simulink model "Control_test"  (R2014b)
settings: Solver=FixedStepDiscrete  StartTime=0.0  StopTime=Inf  FixedStep=0.001  RelTol=1e-3
PostLoadFcn:
  | , if any(exist('dsrtsu_mdlpostloadfcn', 'file') == [2, 3, 6]), try dsrtsu_mdlpostloadfcn('Execute', bdroot); catch fprintf('Error in PostLoadFcn (dsrtsu_mdlpostloadfcn) for model "%s":\n %s\n', bdroot, lasterr); end, end,
undefined symbols (not defined in the file or in its folder): dtLocal, slcm
libraries: rtican x163, simulink x14
(part 33 of 34)

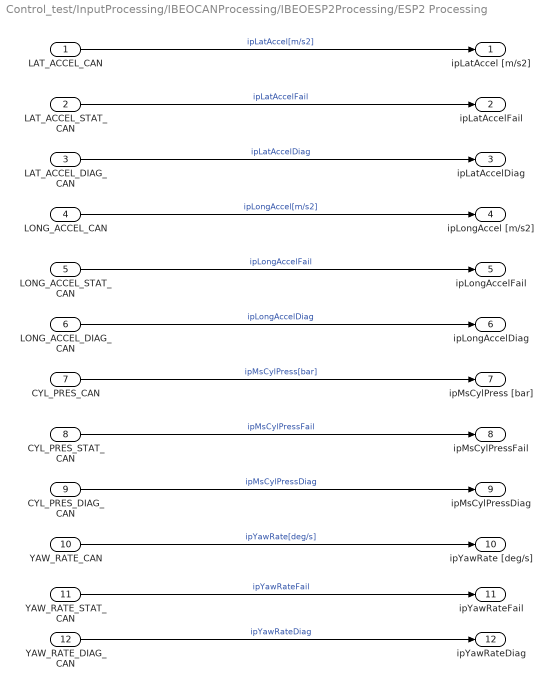
== system Control_test/InputProcessing/IBEOCANProcessing/IBEOESP2Processing/ESP2 Processing ==
  LAT_ACCEL_CAN : Inport
  LAT_ACCEL_STAT_CAN : Inport  Port=2
  LAT_ACCEL_DIAG_CAN : Inport  Port=3
  LONG_ACCEL_CAN : Inport  Port=4
  LONG_ACCEL_STAT_CAN : Inport  Port=5
  LONG_ACCEL_DIAG_CAN : Inport  Port=6
  CYL_PRES_CAN : Inport  Port=7
  CYL_PRES_STAT_CAN : Inport  Port=8
  CYL_PRES_DIAG_CAN : Inport  Port=9
  YAW_RATE_CAN : Inport  Port=10
  YAW_RATE_STAT_CAN : Inport  Port=11
  YAW_RATE_DIAG_CAN : Inport  Port=12
  ipLatAccel [m/s2] : Outport
  ipLatAccelFail : Outport  Port=2
  ipLatAccelDiag : Outport  Port=3
  ipLongAccel [m/s2] : Outport  Port=4
  ipLongAccelFail : Outport  Port=5
  ipLongAccelDiag : Outport  Port=6
  ipMsCylPress [bar] : Outport  Port=7
  ipMsCylPressFail : Outport  Port=8
  ipMsCylPressDiag : Outport  Port=9
  ipYawRate [deg/s] : Outport  Port=10
  ipYawRateFail : Outport  Port=11
  ipYawRateDiag : Outport  Port=12
  wires:
  YAW_RATE_CAN/1 -> ipYawRate [deg/s]/1  "ipYawRate[deg/s]"
  LONG_ACCEL_CAN/1 -> ipLongAccel [m/s2]/1  "ipLongAccel[m/s2]"
  LAT_ACCEL_STAT_CAN/1 -> ipLatAccelFail/1  "ipLatAccelFail"
  LAT_ACCEL_DIAG_CAN/1 -> ipLatAccelDiag/1  "ipLatAccelDiag"
  LONG_ACCEL_STAT_CAN/1 -> ipLongAccelFail/1  "ipLongAccelFail"
  LONG_ACCEL_DIAG_CAN/1 -> ipLongAccelDiag/1  "ipLongAccelDiag"
  CYL_PRES_CAN/1 -> ipMsCylPress [bar]/1  "ipMsCylPress[bar]"
  CYL_PRES_STAT_CAN/1 -> ipMsCylPressFail/1  "ipMsCylPressFail"
  CYL_PRES_DIAG_CAN/1 -> ipMsCylPressDiag/1  "ipMsCylPressDiag"
  YAW_RATE_STAT_CAN/1 -> ipYawRateFail/1  "ipYawRateFail"
  YAW_RATE_DIAG_CAN/1 -> ipYawRateDiag/1  "ipYawRateDiag"
  LAT_ACCEL_CAN/1 -> ipLatAccel [m/s2]/1  "ipLatAccel[m/s2]"

== system Control_test/InputProcessing/IBEOCANProcessing/IBEOSASProcessing/SAS1 Processing ==
  SAS_Angle_CAN : Inport
  SAS_Speed_CAN : Inport  Port=2
  MsgCount_CAN : Inport  Port=3
  CheckSum_CAN : Inport  Port=4
  Add2 : Sum  Inputs=+-
  Compare To Constant1 : simulink/Logic and Bit Operations/Compare To Constant  relop=<=  const=3276.7  OutDataTypeStr=boolean  ZeroCross=off
  Constant6 : Constant  Value=6553.6  SampleTime=Inf
  ErrProcessing1 : Subsystem
  ErrProcessing2 : Subsystem
  Switch1 : Switch  Criteria=u2 > Threshold
  ipStrAng [deg] : Outport
  ipStrAngEr : Outport  Port=2
  ipStrSpd [deg/s] : Outport  Port=3
  ipStrSpdEr : Outport  Port=4
  ipSasCnt : Outport  Port=5
  ipSasCksum : Outport  Port=6
  wires:
  SAS_Speed_CAN/1 -> ErrProcessing1/1(In1)
  Add2/1 -> Switch1/3
  Constant6/1 -> Add2/2
  Compare To Constant1/1 -> Switch1/2
  Switch1/1 -> ipStrAng [deg]/1  "ipStrAng[deg]"
  ErrProcessing2/2(ErrFlag) -> ipStrAngEr/1  "ipStrAngEr"
  ErrProcessing1/2(ErrFlag) -> ipStrSpdEr/1  "ipStrSpdEr"
  ErrProcessing1/1(Data) -> ipStrSpd [deg/s]/1  "ipStrSpd[deg/s]"
  MsgCount_CAN/1 -> ipSasCnt/1  "ipSasCnt"
  CheckSum_CAN/1 -> ipSasCksum/1  "ipSasCksum"
  SAS_Angle_CAN/1 -> ErrProcessing2/1(In1)
  ErrProcessing2/1(Data) -> Compare To Constant1/1, Switch1/1, Add2/1

== system Control_test/InputProcessing/RadarCanProcessing/Primary Target Selection/Default ==
  Bus Creator : BusCreator  Inputs=12
  Constant : Constant  Value=255  SampleTime=0.01
  Out1 : Outport
  wires:
  Bus Creator/1 -> Out1/1  "NoTrack"
  Constant/1 -> Bus Creator/1, Bus Creator/2, Bus Creator/3, Bus Creator/4, Bus Creator/5, Bus Creator/6, Bus Creator/7, Bus Creator/8, Bus Creator/9, Bus Creator/10, Bus Creator/11, Bus Creator/12

== system Control_test/InputProcessing/VehicleCanProcessing/CLU2Processing/CLU2Processing ==
  CF_Clu_TrunSigLh_CAN : Inport
  CF_Clu_TurnSigRh_CAN : Inport  Port=2
  ipCluTurnSigLh : Outport
  ipCluTurnSigRh : Outport  Port=2
  wires:
  CF_Clu_TrunSigLh_CAN/1 -> ipCluTurnSigLh/1  "ipCluTurnSigLh"
  CF_Clu_TurnSigRh_CAN/1 -> ipCluTurnSigRh/1  "ipCluTurnSigRh"

== system Control_test/InputProcessing/VehicleCanProcessing/EMS1Processing/EMS1 Processing ==
  VS_CAN : Inport
  ErrProcessing : Subsystem
  ipEmsVehSpd [kph] : Outport
  ipEmsVehSpdFail : Outport  Port=2
  wires:
  VS_CAN/1 -> ErrProcessing/1(In1)
  ErrProcessing/1(Data) -> ipEmsVehSpd [kph]/1  "ipEmsVehSpd[kph]"
  ErrProcessing/2(ErrFlag) -> ipEmsVehSpdFail/1  "ipEmsVehSpdFail"

== system Control_test/InputProcessing/VehicleCanProcessing/ESP2Processing/ESP2 Processing ==
  LAT_ACCEL_CAN : Inport
  LAT_ACCEL_STAT_CAN : Inport  Port=2
  LAT_ACCEL_DIAG_CAN : Inport  Port=3
  LONG_ACCEL_CAN : Inport  Port=4
  LONG_ACCEL_STAT_CAN : Inport  Port=5
  LONG_ACCEL_DIAG_CAN : Inport  Port=6
  CYL_PRES_CAN : Inport  Port=7
  CYL_PRES_STAT_CAN : Inport  Port=8
  CYL_PRES_DIAG_CAN : Inport  Port=9
  YAW_RATE_CAN : Inport  Port=10
  YAW_RATE_STAT_CAN : Inport  Port=11
  YAW_RATE_DIAG_CAN : Inport  Port=12
  ipLatAccel [m/s2] : Outport
  ipLatAccelFail : Outport  Port=2
  ipLatAccelDiag : Outport  Port=3
  ipLongAccel [m/s2] : Outport  Port=4
  ipLongAccelFail : Outport  Port=5
  ipLongAccelDiag : Outport  Port=6
  ipMsCylPress [bar] : Outport  Port=7
  ipMsCylPressFail : Outport  Port=8
  ipMsCylPressDiag : Outport  Port=9
  ipYawRate [deg/s] : Outport  Port=10
  ipYawRateFail : Outport  Port=11
  ipYawRateDiag : Outport  Port=12
  wires:
  YAW_RATE_CAN/1 -> ipYawRate [deg/s]/1  "ipYawRate[deg/s]"
  LONG_ACCEL_CAN/1 -> ipLongAccel [m/s2]/1  "ipLongAccel[m/s2]"
  LAT_ACCEL_STAT_CAN/1 -> ipLatAccelFail/1  "ipLatAccelFail"
  LAT_ACCEL_DIAG_CAN/1 -> ipLatAccelDiag/1  "ipLatAccelDiag"
  LONG_ACCEL_STAT_CAN/1 -> ipLongAccelFail/1  "ipLongAccelFail"
  LONG_ACCEL_DIAG_CAN/1 -> ipLongAccelDiag/1  "ipLongAccelDiag"
  CYL_PRES_CAN/1 -> ipMsCylPress [bar]/1  "ipMsCylPress[bar]"
  CYL_PRES_STAT_CAN/1 -> ipMsCylPressFail/1  "ipMsCylPressFail"
  CYL_PRES_DIAG_CAN/1 -> ipMsCylPressDiag/1  "ipMsCylPressDiag"
  YAW_RATE_STAT_CAN/1 -> ipYawRateFail/1  "ipYawRateFail"
  YAW_RATE_DIAG_CAN/1 -> ipYawRateDiag/1  "ipYawRateDiag"
  LAT_ACCEL_CAN/1 -> ipLatAccel [m/s2]/1  "ipLatAccel[m/s2]"

== system Control_test/InputProcessing/VehicleCanProcessing/MDPS3Processing/MDPS3 Processing ==
  CR_Mdps_StrColTq_CAN : Inport
  CR_Mdps_ToiUnavail_CAN : Inport  Port=2
  CR_Mdps_ToiActive_CAN : Inport  Port=3
  CR_Mdps_ToiFit_CAN : Inport  Port=4
  CR_Mdps_FailStat_CAN : Inport  Port=5
  ipMdpsStrColTq : Outport
  ipMdpsToiUnavail : Outport  Port=2
  ipMdpsToiActive : Outport  Port=3
  ipMdpsToiFit : Outport  Port=4
  ipMdpsFailStat : Outport  Port=5
  wires:
  CR_Mdps_FailStat_CAN/1 -> ipMdpsFailStat/1  "ipMdpsFailStat"
  CR_Mdps_ToiActive_CAN/1 -> ipMdpsToiActive/1  "ipMdpsToiActive"
  CR_Mdps_ToiUnavail_CAN/1 -> ipMdpsToiUnavail/1  "ipMdpsToiUnavail"
  CR_Mdps_StrColTq_CAN/1 -> ipMdpsStrColTq/1  "ipMdpsStrColTq"
  CR_Mdps_ToiFit_CAN/1 -> ipMdpsToiFit/1  "ipMdpsToiFit"

== system Control_test/InputProcessing/VehicleCanProcessing/SAS1Processing/SAS1 Processing ==
  SAS_Angle_CAN : Inport
  SAS_Speed_CAN : Inport  Port=2
  MsgCount_CAN : Inport  Port=3
  CheckSum_CAN : Inport  Port=4
  Add2 : Sum  Inputs=+-
  Compare To Constant1 : simulink/Logic and Bit Operations/Compare To Constant  relop=<=  const=3276.7  OutDataTypeStr=uint8  ZeroCross=off
  Constant6 : Constant  Value=6553.6  SampleTime=Inf
  ErrProcessing1 : Subsystem
  ErrProcessing2 : Subsystem
  Switch1 : Switch  Criteria=u2 > Threshold
  ipStrAng [deg] : Outport
  ipStrAngEr : Outport  Port=2
  ipStrSpd [deg/s] : Outport  Port=3
  ipStrSpdEr : Outport  Port=4
  ipSasCnt : Outport  Port=5
  ipSasCksum : Outport  Port=6
  wires:
  SAS_Speed_CAN/1 -> ErrProcessing1/1(In1)
  Add2/1 -> Switch1/3
  Constant6/1 -> Add2/2
  Compare To Constant1/1 -> Switch1/2
  Switch1/1 -> ipStrAng [deg]/1  "ipStrAng[deg]"
  ErrProcessing2/2(ErrFlag) -> ipStrAngEr/1  "ipStrAngEr"
  ErrProcessing1/2(ErrFlag) -> ipStrSpdEr/1  "ipStrSpdEr"
  ErrProcessing1/1(Data) -> ipStrSpd [deg/s]/1  "ipStrSpd[deg/s]"
  MsgCount_CAN/1 -> ipSasCnt/1  "ipSasCnt"
  CheckSum_CAN/1 -> ipSasCksum/1  "ipSasCksum"
  SAS_Angle_CAN/1 -> ErrProcessing2/1(In1)
  ErrProcessing2/1(Data) -> Compare To Constant1/1, Switch1/1, Add2/1

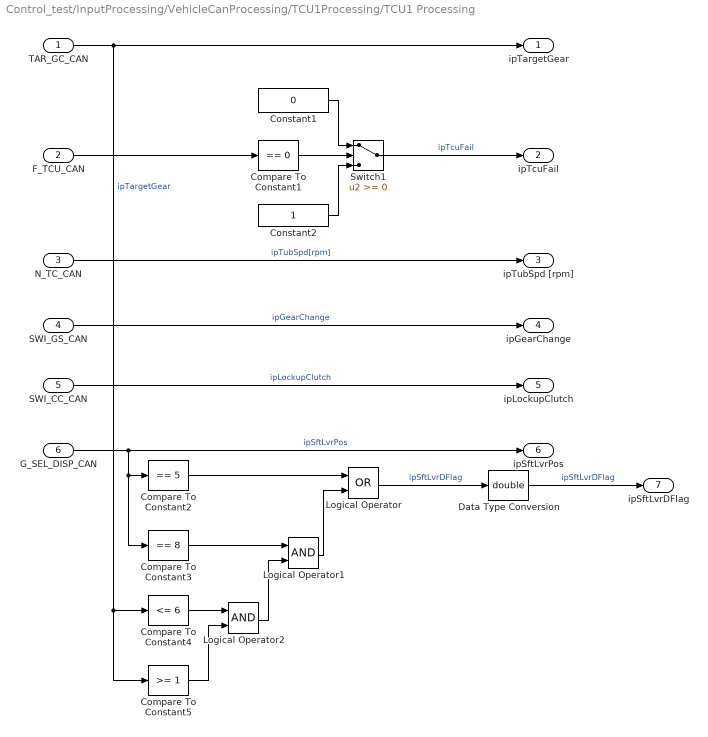
== system Control_test/InputProcessing/VehicleCanProcessing/TCU1Processing/TCU1 Processing ==
  TAR_GC_CAN : Inport
  F_TCU_CAN : Inport  Port=2
  N_TC_CAN : Inport  Port=3
  SWI_GS_CAN : Inport  Port=4
  SWI_CC_CAN : Inport  Port=5
  G_SEL_DISP_CAN : Inport  Port=6
  Compare To Constant1 : simulink/Logic and Bit Operations/Compare To Constant  relop===  const=0  OutDataTypeStr=uint8  ZeroCross=off
  Compare To Constant2 : simulink/Logic and Bit Operations/Compare To Constant  relop===  const=5  OutDataTypeStr=uint8  ZeroCross=off
  Compare To Constant3 : simulink/Logic and Bit Operations/Compare To Constant  relop===  const=8  OutDataTypeStr=uint8  ZeroCross=off
  Compare To Constant4 : simulink/Logic and Bit Operations/Compare To Constant  relop=<=  const=6  OutDataTypeStr=uint8  ZeroCross=off
  Compare To Constant5 : simulink/Logic and Bit Operations/Compare To Constant  relop=>=  const=1  OutDataTypeStr=uint8  ZeroCross=off
  Constant1 : Constant  Value=0  SampleTime=Inf
  Constant2 : Constant  SampleTime=Inf
  Data Type Conversion : DataTypeConversion  OutDataTypeStr=double
  Logical Operator : Logic  Operator=OR  AllPortsSameDT=off  OutDataTypeStr=boolean
  Logical Operator1 : Logic  AllPortsSameDT=off  OutDataTypeStr=boolean
  Logical Operator2 : Logic  AllPortsSameDT=off  OutDataTypeStr=boolean
  Switch1 : Switch
  ipTargetGear : Outport
  ipTcuFail : Outport  Port=2
  ipTubSpd [rpm] : Outport  Port=3
  ipGearChange : Outport  Port=4
  ipLockupClutch : Outport  Port=5
  ipSftLvrPos : Outport  Port=6
  ipSftLvrDFlag : Outport  Port=7
  wires:
  Compare To Constant5/1 -> Logical Operator2/2
  Logical Operator2/1 -> Logical Operator1/2
  Compare To Constant4/1 -> Logical Operator2/1
  Logical Operator1/1 -> Logical Operator/2
  Compare To Constant3/1 -> Logical Operator1/1
  Logical Operator/1 -> Data Type Conversion/1  "ipSftLvrDFlag"
  Compare To Constant2/1 -> Logical Operator/1
  G_SEL_DISP_CAN/1 -> Compare To Constant3/1, Compare To Constant2/1, ipSftLvrPos/1  "ipSftLvrPos"
  SWI_CC_CAN/1 -> ipLockupClutch/1  "ipLockupClutch"
  SWI_GS_CAN/1 -> ipGearChange/1  "ipGearChange"
  N_TC_CAN/1 -> ipTubSpd [rpm]/1  "ipTubSpd[rpm]"
  Switch1/1 -> ipTcuFail/1  "ipTcuFail"
  Constant2/1 -> Switch1/3
  Constant1/1 -> Switch1/1
  Compare To Constant1/1 -> Switch1/2
  F_TCU_CAN/1 -> Compare To Constant1/1
  TAR_GC_CAN/1 -> Compare To Constant5/1, Compare To Constant4/1, ipTargetGear/1  "ipTargetGear"
  Data Type Conversion/1 -> ipSftLvrDFlag/1  "ipSftLvrDFlag"

== system Control_test/InputProcessing/VehicleCanProcessing/WhlSpdProcessing/WhlSpd Processing ==
  WHL_SPD_FL_CAN : Inport
  WHL_SPD_FR_CAN : Inport  Port=2
  WHL_SPD_RL_CAN : Inport  Port=3
  WHL_SPD_RR_CAN : Inport  Port=4
  Add2 : Sum
  Constant3 : Constant  Value=2  SampleTime=Inf
  ErrProcessing : Subsystem
  ErrProcessing1 : Subsystem
  ErrProcessing2 : Subsystem
  ErrProcessing3 : Subsystem
  Gain : Gain  Gain=1/3.6
  Product5 : Product  Inputs=*/
  ipWhlSpdFl [kph] : Outport
  ipWhlSpdFlEr : Outport  Port=2
  ipWhlSpdFr [kph] : Outport  Port=3
  ipWhlSpdFrEr : Outport  Port=4
  ipWhlSpdRl [kph] : Outport  Port=5
  ipWhlSpdRlEr : Outport  Port=6
  ipWhlSpdRr [kph] : Outport  Port=7
  ipWhlSpdRrEr : Outport  Port=8
  ipVehSpdWhl [kph] : Outport  Port=9
  ipVehSpdWhl [m/s] : Outport  Port=10
  wires:
  Gain/1 -> ipVehSpdWhl [m/s]/1  "ipVehSpdWhl[m/s]"
  Constant3/1 -> Product5/2
  Add2/1 -> Product5/1
  WHL_SPD_FR_CAN/1 -> ErrProcessing1/1(In1)
  WHL_SPD_FL_CAN/1 -> ErrProcessing/1(In1)
  ErrProcessing/1(Data) -> Add2/1, ipWhlSpdFl [kph]/1  "ipWhlSpdFl[kph]"
  ErrProcessing/2(ErrFlag) -> ipWhlSpdFlEr/1  "ipWhlSpdFlEr"
  ErrProcessing1/1(Data) -> Add2/2, ipWhlSpdFr [kph]/1  "ipWhlSpdFr[kph]"
  ErrProcessing1/2(ErrFlag) -> ipWhlSpdFrEr/1  "ipWhlSpdFrEr"
  WHL_SPD_RL_CAN/1 -> ErrProcessing2/1(In1)
  ErrProcessing2/1(Data) -> ipWhlSpdRl [kph]/1  "ipWhlSpdRl[kph]"
  ErrProcessing2/2(ErrFlag) -> ipWhlSpdRlEr/1  "ipWhlSpdRlEr"
  WHL_SPD_RR_CAN/1 -> ErrProcessing3/1(In1)
  ErrProcessing3/1(Data) -> ipWhlSpdRr [kph]/1  "ipWhlSpdRr[kph]"
  ErrProcessing3/2(ErrFlag) -> ipWhlSpdRrEr/1  "ipWhlSpdRrEr"
  Product5/1 -> ipVehSpdWhl [kph]/1, Gain/1  "ipVehSpdWhl[kph]"

== system Control_test/OutputProcessing/RadarCanProcessing/Transmit Radar Msg 0x4F0/If Action Subsystem ==
  In1 : Inport
  Action Port : ActionPort  ActionType=then
  Out1 : Outport
  wires:
  In1/1 -> Out1/1

== system Control_test/OutputProcessing/RadarCanProcessing/Transmit Radar Msg 0x4F0/If Action Subsystem1 ==
  In1 : Inport
  Action Port : ActionPort  ActionType=else
  Out1 : Outport
  wires:
  In1/1 -> Out1/1

== system Control_test/OutputProcessing/VehicleCanProcessing/LKAS2/Angle 2 Torque ==
  ISAS_Cmd(deg) : Inport
  ControlOn : Inport  Port=2
  Vs : Inport  Port=3
  SteeringAngle : Inport  Port=4
  IGainSpeed : Gain
  I_gain_spd : Constant  Value=500
  PGainSAS : Gain
  PGainSpeed : Gain
  PI controller : Subsystem
  P_gain_sas_map : Lookup  InputValues=[0,30,60,80,100]  Table=[170,170,300,300,330]  LookUpMeth=Interpolation-Use End Values
  P_gain_spd_map : Lookup  InputValues=[0,30,60,80,100]  Table=[300,300,400,400,450]  LookUpMeth=Interpolation-Use End Values
  Rate Limiter steering : RateLimiter  RisingSlewLimit=50  FallingSlewLimit=-50  SampleTimeMode=inherited
  Saturation steering torque : Saturate  UpperLimit=7.5  LowerLimit=-7.5
  Steering TQ : Outport
  wires:
  I_gain_spd/1 -> IGainSpeed/1
  ControlOn/1 -> PI controller/1(Active_flag)  "ActiveFlag"
  ISAS_Cmd(deg)/1 -> PI controller/2(SAS_Cmd(deg))  "SAS_Cmd"
  SteeringAngle/1 -> PI controller/3(SAS_Angle(deg))
  Saturation steering torque/1 -> Rate Limiter steering/1  "Tq_after_sat"
  Rate Limiter steering/1 -> Steering TQ/1  "Control Tq"
  Vs/1 -> P_gain_spd_map/1, P_gain_sas_map/1
  PI controller/1(Tq) -> Saturation steering torque/1  "Tq_before_sat"
  P_gain_sas_map/1 -> PGainSAS/1
  P_gain_spd_map/1 -> PGainSpeed/1
  PGainSpeed/1 -> PI controller/5(P_gain_spd)  "PGainSpeed"
  PGainSAS/1 -> PI controller/4(P_gain_sas)  "PGainSAS"
  IGainSpeed/1 -> PI controller/6(I_gain_spd)

== system Control_test/OutputProcessing/VehicleCanProcessing/LKAS2/TxLKAS2CAN ==
  Tq : Inport
  ActiveFlag_Out : Inport  Port=2
  TOI_Fault : Inport  Port=3
  MessageCounter : Subsystem  mask(Rolling Counter){cyc_time=20, calc_time=2, n_bit=4}
      mask prompts: cyc_time "Cyclic Time (ms)"; calc_time "Model loop time [ms]"; n_bit "Number of bits"
      mask help: This block is a rolling counter that overflows back to zero after it has been the maximum value for the specified number of bits.
  Tx_ADAS_data : Subsystem
  Checksum_Out : Outport
  LKAS_Tq_Out : Outport  Port=2
  MessageCounter_Out : Outport  Port=3
  TOI_Fault_Out : Outport  Port=4
  ActiveTOI_Out : Outport  Port=5
  wires:
  MessageCounter/1(Counter) -> Tx_ADAS_data/1(MessageCounter)
  Tx_ADAS_data/1(LKAS_Toq_Out) -> LKAS_Tq_Out/1
  Tq/1 -> Tx_ADAS_data/2(SteeringTorqueRuest)
  ActiveFlag_Out/1 -> Tx_ADAS_data/3(ActiveTOI)
  Tx_ADAS_data/4(MessageCounter_Out) -> MessageCounter_Out/1
  Tx_ADAS_data/2(ActiveTOI_Out) -> ActiveTOI_Out/1
  TOI_Fault/1 -> Tx_ADAS_data/4(TOI_Fault)
  Tx_ADAS_data/3(TOI_Fault_Out) -> TOI_Fault_Out/1
  Tx_ADAS_data/5(Checksum_Out) -> Checksum_Out/1

== system Control_test/RTI Data/RTI Data Store/RTI Data Store/RTI Data Store ==
  RTI Data Store : Subsystem  mask(RTI_DATA_STORE){}
      mask help:
      | RTI Data Store Block. This block is used by RTI to store internal model dependent data. Deleting this block will result in data loss.
      |
      | NEVER DELETE, COPY, OR MODIFY THIS BLOCK!
      mask Help:
      | RTI Data Store Block. This block is used by RTI to store internal model dependent data. Deleting this block will result in data loss.
      | 
      | NEVER DELETE, COPY, OR MODIFY THIS BLOCK!
      mask Display: text(0.5, 0.5, ' ', 'HorizontalAlignment', 'center');

== system Control_test/InputProcessing/IBEOCANProcessing/IBEOSASProcessing/SAS1 Processing/ErrProcessing1 ==
  In1 : Inport
  If : If  NumInputs=2  IfExpression=u1 == 1020 & u2>1  ElseIfExpressions=u1 == 1020 & u2<=1
  If Action Subsystem : Subsystem  TreatAsAtomicUnit=on
  If Action Subsystem1 : Subsystem  TreatAsAtomicUnit=on
  If Action Subsystem2 : Subsystem  TreatAsAtomicUnit=on
  Memory : Memory
  Memory1 : Memory
  Merge : Merge  Inputs=3
  Merge1 : Merge  Inputs=3
  Merge2 : Merge  Inputs=3
  Data : Outport
  ErrFlag : Outport  Port=2
  wires:
  In1/1 -> If/1, If Action Subsystem1/1(In1)
  If/1 -> If Action Subsystem/Action
  If/3 -> If Action Subsystem1/Action
  If/2 -> If Action Subsystem2/Action
  If Action Subsystem/1(Data) -> Merge/1
  If Action Subsystem2/1(Data) -> Merge/2
  If Action Subsystem1/1(Data) -> Merge/3
  Merge/1 -> Data/1, Memory1/1
  Memory1/1 -> If Action Subsystem2/1(In1)
  If Action Subsystem/2(Count) -> Merge1/1
  If Action Subsystem2/2(Count) -> Merge1/2
  If Action Subsystem1/2(Count) -> Merge1/3
  Merge1/1 -> Memory/1
  Memory/1 -> If Action Subsystem/1(In1), If/2, If Action Subsystem2/2(In2)
  If Action Subsystem/3(Flag) -> Merge2/1
  If Action Subsystem2/3(Flag) -> Merge2/2
  If Action Subsystem1/3(Flag) -> Merge2/3
  Merge2/1 -> ErrFlag/1

== system Control_test/InputProcessing/IBEOCANProcessing/IBEOSASProcessing/SAS1 Processing/ErrProcessing2 ==
  In1 : Inport
  If : If  NumInputs=2  IfExpression=u1 == 3276.7 & u2>1  ElseIfExpressions=u1 == 3276.7 & u2<=1
  If Action Subsystem : Subsystem  TreatAsAtomicUnit=on
  If Action Subsystem1 : Subsystem  TreatAsAtomicUnit=on
  If Action Subsystem2 : Subsystem  TreatAsAtomicUnit=on
  Memory : Memory
  Memory1 : Memory
  Merge : Merge  Inputs=3
  Merge1 : Merge  Inputs=3
  Merge2 : Merge  Inputs=3
  Data : Outport
  ErrFlag : Outport  Port=2
  wires:
  Merge2/1 -> ErrFlag/1
  If Action Subsystem1/3(Flag) -> Merge2/3
  If Action Subsystem2/3(Flag) -> Merge2/2
  If Action Subsystem/3(Flag) -> Merge2/1
  Memory/1 -> If Action Subsystem2/2(In2), If/2, If Action Subsystem/1(In1)
  Merge1/1 -> Memory/1
  If Action Subsystem1/2(Count) -> Merge1/3
  If Action Subsystem2/2(Count) -> Merge1/2
  If Action Subsystem/2(Count) -> Merge1/1
  Memory1/1 -> If Action Subsystem2/1(In1)
  Merge/1 -> Memory1/1, Data/1
  If Action Subsystem1/1(Data) -> Merge/3
  If Action Subsystem2/1(Data) -> Merge/2
  If Action Subsystem/1(Data) -> Merge/1
  If/2 -> If Action Subsystem2/Action
  If/3 -> If Action Subsystem1/Action
  If/1 -> If Action Subsystem/Action
  In1/1 -> If Action Subsystem1/1(In1), If/1

== system Control_test/InputProcessing/VehicleCanProcessing/EMS1Processing/EMS1 Processing/ErrProcessing ==
  In1 : Inport
  If : If  NumInputs=2  IfExpression=u1 == 255 & u2>1  ElseIfExpressions=u1 == 255 & u2<=1
  If Action Subsystem : Subsystem  TreatAsAtomicUnit=on
  If Action Subsystem1 : Subsystem  TreatAsAtomicUnit=on
  If Action Subsystem2 : Subsystem  TreatAsAtomicUnit=on
  Memory : Memory
  Memory1 : Memory
  Merge : Merge  Inputs=3
  Merge1 : Merge  Inputs=3
  Merge2 : Merge  Inputs=3
  Data : Outport
  ErrFlag : Outport  Port=2
  wires:
  In1/1 -> If/1, If Action Subsystem1/1(In1)
  If/1 -> If Action Subsystem/Action
  If/3 -> If Action Subsystem1/Action
  If/2 -> If Action Subsystem2/Action
  If Action Subsystem/1(Data) -> Merge/1
  If Action Subsystem2/1(Data) -> Merge/2
  If Action Subsystem1/1(Data) -> Merge/3
  Merge/1 -> Data/1, Memory1/1
  Memory1/1 -> If Action Subsystem2/1(In1)
  If Action Subsystem/2(Count) -> Merge1/1
  If Action Subsystem2/2(Count) -> Merge1/2
  If Action Subsystem1/2(Count) -> Merge1/3
  Merge1/1 -> Memory/1
  Memory/1 -> If Action Subsystem/1(In1), If/2, If Action Subsystem2/2(In2)
  If Action Subsystem/3(Flag) -> Merge2/1
  If Action Subsystem2/3(Flag) -> Merge2/2
  If Action Subsystem1/3(Flag) -> Merge2/3
  Merge2/1 -> ErrFlag/1

== system Control_test/InputProcessing/VehicleCanProcessing/SAS1Processing/SAS1 Processing/ErrProcessing1 ==
  In1 : Inport
  If : If  NumInputs=2  IfExpression=u1 == 1020 & u2>1  ElseIfExpressions=u1 == 1020 & u2<=1
  If Action Subsystem : Subsystem  TreatAsAtomicUnit=on
  If Action Subsystem1 : Subsystem  TreatAsAtomicUnit=on
  If Action Subsystem2 : Subsystem  TreatAsAtomicUnit=on
  Memory : Memory
  Memory1 : Memory
  Merge : Merge  Inputs=3
  Merge1 : Merge  Inputs=3
  Merge2 : Merge  Inputs=3
  Data : Outport
  ErrFlag : Outport  Port=2
  wires:
  In1/1 -> If/1, If Action Subsystem1/1(In1)
  If/1 -> If Action Subsystem/Action
  If/3 -> If Action Subsystem1/Action
  If/2 -> If Action Subsystem2/Action
  If Action Subsystem/1(Data) -> Merge/1
  If Action Subsystem2/1(Data) -> Merge/2
  If Action Subsystem1/1(Data) -> Merge/3
  Merge/1 -> Data/1, Memory1/1
  Memory1/1 -> If Action Subsystem2/1(In1)
  If Action Subsystem/2(Count) -> Merge1/1
  If Action Subsystem2/2(Count) -> Merge1/2
  If Action Subsystem1/2(Count) -> Merge1/3
  Merge1/1 -> Memory/1
  Memory/1 -> If Action Subsystem/1(In1), If/2, If Action Subsystem2/2(In2)
  If Action Subsystem/3(Flag) -> Merge2/1
  If Action Subsystem2/3(Flag) -> Merge2/2
  If Action Subsystem1/3(Flag) -> Merge2/3
  Merge2/1 -> ErrFlag/1

== system Control_test/InputProcessing/VehicleCanProcessing/SAS1Processing/SAS1 Processing/ErrProcessing2 ==
  In1 : Inport
  If : If  NumInputs=2  IfExpression=u1 == 3276.7 & u2>1  ElseIfExpressions=u1 == 3276.7 & u2<=1
  If Action Subsystem : Subsystem  TreatAsAtomicUnit=on
  If Action Subsystem1 : Subsystem  TreatAsAtomicUnit=on
  If Action Subsystem2 : Subsystem  TreatAsAtomicUnit=on
  Memory : Memory
  Memory1 : Memory
  Merge : Merge  Inputs=3
  Merge1 : Merge  Inputs=3
  Merge2 : Merge  Inputs=3
  Data : Outport
  ErrFlag : Outport  Port=2
  wires:
  Merge2/1 -> ErrFlag/1
  If Action Subsystem1/3(Flag) -> Merge2/3
  If Action Subsystem2/3(Flag) -> Merge2/2
  If Action Subsystem/3(Flag) -> Merge2/1
  Memory/1 -> If Action Subsystem2/2(In2), If/2, If Action Subsystem/1(In1)
  Merge1/1 -> Memory/1
  If Action Subsystem1/2(Count) -> Merge1/3
  If Action Subsystem2/2(Count) -> Merge1/2
  If Action Subsystem/2(Count) -> Merge1/1
  Memory1/1 -> If Action Subsystem2/1(In1)
  Merge/1 -> Memory1/1, Data/1
  If Action Subsystem1/1(Data) -> Merge/3
  If Action Subsystem2/1(Data) -> Merge/2
  If Action Subsystem/1(Data) -> Merge/1
  If/2 -> If Action Subsystem2/Action
  If/3 -> If Action Subsystem1/Action
  If/1 -> If Action Subsystem/Action
  In1/1 -> If Action Subsystem1/1(In1), If/1

== system Control_test/InputProcessing/VehicleCanProcessing/WhlSpdProcessing/WhlSpd Processing/ErrProcessing ==
  In1 : Inport
  If : If  NumInputs=2  IfExpression=u1 == 511.96875 & u2>1  ElseIfExpressions=u1 == 511.96875 & u2<=1
  If Action Subsystem : Subsystem  TreatAsAtomicUnit=on
  If Action Subsystem1 : Subsystem  TreatAsAtomicUnit=on
  If Action Subsystem2 : Subsystem  TreatAsAtomicUnit=on
  Memory : Memory
  Memory1 : Memory
  Merge : Merge  Inputs=3
  Merge1 : Merge  Inputs=3
  Merge2 : Merge  Inputs=3
  Data : Outport
  ErrFlag : Outport  Port=2
  wires:
  In1/1 -> If/1, If Action Subsystem1/1(In1)
  If/1 -> If Action Subsystem/Action
  If/3 -> If Action Subsystem1/Action
  If/2 -> If Action Subsystem2/Action
  If Action Subsystem/1(Data) -> Merge/1
  If Action Subsystem2/1(Data) -> Merge/2
  If Action Subsystem1/1(Data) -> Merge/3
  Merge/1 -> Data/1, Memory1/1
  Memory1/1 -> If Action Subsystem2/1(In1)
  If Action Subsystem/2(Count) -> Merge1/1
  If Action Subsystem2/2(Count) -> Merge1/2
  If Action Subsystem1/2(Count) -> Merge1/3
  Merge1/1 -> Memory/1
  Memory/1 -> If Action Subsystem/1(In1), If/2, If Action Subsystem2/2(In2)
  If Action Subsystem/3(Flag) -> Merge2/1
  If Action Subsystem2/3(Flag) -> Merge2/2
  If Action Subsystem1/3(Flag) -> Merge2/3
  Merge2/1 -> ErrFlag/1

== system Control_test/InputProcessing/VehicleCanProcessing/WhlSpdProcessing/WhlSpd Processing/ErrProcessing1 ==
  In1 : Inport
  If : If  NumInputs=2  IfExpression=u1 == 511.96875 & u2>1  ElseIfExpressions=u1 == 511.96875 & u2<=1
  If Action Subsystem : Subsystem  TreatAsAtomicUnit=on
  If Action Subsystem1 : Subsystem  TreatAsAtomicUnit=on
  If Action Subsystem2 : Subsystem  TreatAsAtomicUnit=on
  Memory : Memory
  Memory1 : Memory
  Merge : Merge  Inputs=3
  Merge1 : Merge  Inputs=3
  Merge2 : Merge  Inputs=3
  Data : Outport
  ErrFlag : Outport  Port=2
  wires:
  Merge2/1 -> ErrFlag/1
  If Action Subsystem1/3(Flag) -> Merge2/3
  If Action Subsystem2/3(Flag) -> Merge2/2
  If Action Subsystem/3(Flag) -> Merge2/1
  Memory/1 -> If Action Subsystem2/2(In2), If/2, If Action Subsystem/1(In1)
  Merge1/1 -> Memory/1
  If Action Subsystem1/2(Count) -> Merge1/3
  If Action Subsystem2/2(Count) -> Merge1/2
  If Action Subsystem/2(Count) -> Merge1/1
  Memory1/1 -> If Action Subsystem2/1(In1)
  Merge/1 -> Memory1/1, Data/1
  If Action Subsystem1/1(Data) -> Merge/3
  If Action Subsystem2/1(Data) -> Merge/2
  If Action Subsystem/1(Data) -> Merge/1
  If/2 -> If Action Subsystem2/Action
  If/3 -> If Action Subsystem1/Action
  If/1 -> If Action Subsystem/Action
  In1/1 -> If Action Subsystem1/1(In1), If/1

== system Control_test/InputProcessing/VehicleCanProcessing/WhlSpdProcessing/WhlSpd Processing/ErrProcessing2 ==
  In1 : Inport
  If : If  NumInputs=2  IfExpression=u1 == 511.96875 & u2>1  ElseIfExpressions=u1 == 511.96875 & u2<=1
  If Action Subsystem : Subsystem  TreatAsAtomicUnit=on
  If Action Subsystem1 : Subsystem  TreatAsAtomicUnit=on
  If Action Subsystem2 : Subsystem  TreatAsAtomicUnit=on
  Memory : Memory
  Memory1 : Memory
  Merge : Merge  Inputs=3
  Merge1 : Merge  Inputs=3
  Merge2 : Merge  Inputs=3
  Data : Outport
  ErrFlag : Outport  Port=2
  wires:
  In1/1 -> If/1, If Action Subsystem1/1(In1)
  If/1 -> If Action Subsystem/Action
  If/3 -> If Action Subsystem1/Action
  If/2 -> If Action Subsystem2/Action
  If Action Subsystem/1(Data) -> Merge/1
  If Action Subsystem2/1(Data) -> Merge/2
  If Action Subsystem1/1(Data) -> Merge/3
  Merge/1 -> Data/1, Memory1/1
  Memory1/1 -> If Action Subsystem2/1(In1)
  If Action Subsystem/2(Count) -> Merge1/1
  If Action Subsystem2/2(Count) -> Merge1/2
  If Action Subsystem1/2(Count) -> Merge1/3
  Merge1/1 -> Memory/1
  Memory/1 -> If Action Subsystem/1(In1), If/2, If Action Subsystem2/2(In2)
  If Action Subsystem/3(Flag) -> Merge2/1
  If Action Subsystem2/3(Flag) -> Merge2/2
  If Action Subsystem1/3(Flag) -> Merge2/3
  Merge2/1 -> ErrFlag/1

== system Control_test/InputProcessing/VehicleCanProcessing/WhlSpdProcessing/WhlSpd Processing/ErrProcessing3 ==
  In1 : Inport
  If : If  NumInputs=2  IfExpression=u1 == 511.96875 & u2>1  ElseIfExpressions=u1 == 511.96875 & u2<=1
  If Action Subsystem : Subsystem  TreatAsAtomicUnit=on
  If Action Subsystem1 : Subsystem  TreatAsAtomicUnit=on
  If Action Subsystem2 : Subsystem  TreatAsAtomicUnit=on
  Memory : Memory
  Memory1 : Memory
  Merge : Merge  Inputs=3
  Merge1 : Merge  Inputs=3
  Merge2 : Merge  Inputs=3
  Data : Outport
  ErrFlag : Outport  Port=2
  wires:
  Merge2/1 -> ErrFlag/1
  If Action Subsystem1/3(Flag) -> Merge2/3
  If Action Subsystem2/3(Flag) -> Merge2/2
  If Action Subsystem/3(Flag) -> Merge2/1
  Memory/1 -> If Action Subsystem2/2(In2), If/2, If Action Subsystem/1(In1)
  Merge1/1 -> Memory/1
  If Action Subsystem1/2(Count) -> Merge1/3
  If Action Subsystem2/2(Count) -> Merge1/2
  If Action Subsystem/2(Count) -> Merge1/1
  Memory1/1 -> If Action Subsystem2/1(In1)
  Merge/1 -> Memory1/1, Data/1
  If Action Subsystem1/1(Data) -> Merge/3
  If Action Subsystem2/1(Data) -> Merge/2
  If Action Subsystem/1(Data) -> Merge/1
  If/2 -> If Action Subsystem2/Action
  If/3 -> If Action Subsystem1/Action
  If/1 -> If Action Subsystem/Action
  In1/1 -> If Action Subsystem1/1(In1), If/1

== system Control_test/OutputProcessing/VehicleCanProcessing/LKAS2/Angle 2 Torque/PI controller ==
  Active_flag : Inport
  SAS_Cmd(deg) : Inport  Port=2
  SAS_Angle(deg) : Inport  Port=3
  P_gain_sas : Inport  Port=4
  P_gain_spd : Inport  Port=5
  I_gain_spd : Inport  Port=6
  Product2 : Product  RndMeth=Zero
  SAS_Control : Subsystem  TreatAsAtomicUnit=on
  SAS_Speed_Control : Subsystem
  Tq : Outport
  wires:
  [Active_Flag] -> Product2/2
  [SAS_Cmd] -> SAS_Control/1(SAS_Cmd)
  [SAS_Angle] -> SAS_Control/2(SAS)
  [Active_Flag] -> SAS_Control/3(ActiveFlag)
  SAS_Control/1(SAS_Speed_error) -> SAS_Speed_Control/1(speed err)
  SAS_Speed_Control/1(Out1) -> Product2/1
  [Active_Flag] -> SAS_Speed_Control/4(Active_Flag)
  Product2/1 -> Tq/1
  SAS_Cmd(deg)/1 -> [SAS_Cmd]
  SAS_Angle(deg)/1 -> [SAS_Angle]
  Active_flag/1 -> [Active_Flag]
  P_gain_sas/1 -> [P_gain_sas]
  P_gain_spd/1 -> [P_gain_spd]
  I_gain_spd/1 -> [I_gain_spd]
  [P_gain_spd] -> SAS_Speed_Control/2(P_gain_spd1)
  [I_gain_spd] -> SAS_Speed_Control/3(I_gain_spd1)
  [P_gain_sas] -> SAS_Control/4(P_gain_sas1)

== system Control_test/OutputProcessing/VehicleCanProcessing/LKAS2/TxLKAS2CAN/MessageCounter ==
  note: 1. Trigger Signal out per every cyclic time (ms)
      |
      | 2. Count that overflows back to zero after it has been the maximum value for the specified number of bits.
  note: Rolling Counter
      | Grade of Modification : Low
  Calc. Time (ms) : Constant  Value=calc_time
  Cycle Time (ms) : Constant  Value=cyc_time
  Data Type Conversion : DataTypeConversion  OutDataTypeStr=double
  Data Type Conversion1 : DataTypeConversion  OutDataTypeStr=double
  Divide : Product  Inputs=*/
  Increment : Constant
  Max Value : Constant  Value=2 ^ (n_bit)
  Relational Operator : RelationalOperator  InputSameDT=on
  Relational Operator2 : RelationalOperator  InputSameDT=on
  Reset Value : Constant  Value=0
  Reset Value1 : Constant  Value=0
  "Shinho Systems Co., Ltd." : Subsystem
      mask Display: text( 5,40 , 'Rolling Counter')
  Sum : Sum  SaturateOnIntegerOverflow=on  InputSameDT=on  OutDataTypeStr=Inherit: Same as first input
  Sum1 : Sum  SaturateOnIntegerOverflow=on  InputSameDT=on  OutDataTypeStr=Inherit: Same as first input
  Switch : Switch  Criteria=u2 ~= 0  SaturateOnIntegerOverflow=on  InputSameDT=on
  Switch2 : Switch  Criteria=u2 ~= 0  SaturateOnIntegerOverflow=on  InputSameDT=on
  Unit Delay : UnitDelay  SampleTime=-1
  Unit Delay1 : UnitDelay  SampleTime=-1
  Counter : Outport
  wires:
  Divide/1 -> Relational Operator/2
  Calc. Time (ms)/1 -> Divide/2
  Cycle Time (ms)/1 -> Divide/1
  Data Type Conversion1/1 -> Counter/1  "Counter"
  Unit Delay1/1 -> Sum1/1, Data Type Conversion1/1
  Unit Delay/1 -> Sum/1
  Increment/1 -> Sum/2
  Data Type Conversion/1 -> Sum1/2
  Max Value/1 -> Relational Operator2/2
  Sum1/1 -> Switch2/3, Relational Operator2/1
  Relational Operator2/1 -> Switch2/2
  Reset Value1/1 -> Switch2/1
  Switch2/1 -> Unit Delay1/1
  Sum/1 -> Switch/3, Relational Operator/1
  Relational Operator/1 -> Data Type Conversion/1, Switch/2
  Reset Value/1 -> Switch/1
  Switch/1 -> Unit Delay/1

== system Control_test/OutputProcessing/VehicleCanProcessing/LKAS2/TxLKAS2CAN/Tx_ADAS_data ==
  MessageCounter : Inport
  SteeringTorqueRuest : Inport  Port=2
  ActiveTOI : Inport  Port=3
  TOI_Fault : Inport  Port=4
  Checksum_NEW : Subsystem
  Data Type Conversion{1..2,9,11..12,14} (6 alike) : DataTypeConversion
  LKAS_Toq_Out : Outport
  ActiveTOI_Out : Outport  Port=2
  TOI_Fault_Out : Outport  Port=3
  MessageCounter_Out : Outport  Port=4
  Checksum_Out : Outport  Port=5
  wires:
  Data Type Conversion1/1 -> Data Type Conversion12/1, Checksum_NEW/4(MessageCount)  "MessageCounter"
  TOI_Fault/1 -> Data Type Conversion11/1, Checksum_NEW/3(TOI_Fault)
  MessageCounter/1 -> Data Type Conversion1/1
  Data Type Conversion12/1 -> MessageCounter_Out/1  "MessageCounter"
  Data Type Conversion9/1 -> ActiveTOI_Out/1  "ActiveFlag"
  SteeringTorqueRuest/1 -> Checksum_NEW/1(SteeringTorqueRequest), Data Type Conversion2/1
  ActiveTOI/1 -> Data Type Conversion9/1, Checksum_NEW/2(Active_TOI)
  Data Type Conversion2/1 -> LKAS_Toq_Out/1  "LKAS_Toq"
  Data Type Conversion11/1 -> TOI_Fault_Out/1
  Checksum_NEW/1(Checksum_Out) -> Data Type Conversion14/1
  Data Type Conversion14/1 -> Checksum_Out/1  "Checksum_Out"

== system Control_test/RTI Data/RTI Data Store/RTI Data Store/RTI Data Store/RTI Data Store ==

== system Control_test/InputProcessing/IBEOCANProcessing/IBEOSASProcessing/SAS1 Processing/ErrProcessing1/If Action Subsystem ==
  In1 : Inport
  Action Port : ActionPort  ActionType=then
  Constant : Constant  Value=0
  Constant1 : Constant
  Data : Outport
  Count : Outport  Port=2
  Flag : Outport  Port=3
  wires:
  Constant1/1 -> Flag/1
  In1/1 -> Count/1
  Constant/1 -> Data/1

== system Control_test/InputProcessing/IBEOCANProcessing/IBEOSASProcessing/SAS1 Processing/ErrProcessing1/If Action Subsystem1 ==
  In1 : Inport
  Action Port : ActionPort  ActionType=else
  Constant : Constant  Value=0
  Constant1 : Constant  Value=0
  Data : Outport
  Count : Outport  Port=2
  Flag : Outport  Port=3
  wires:
  Constant1/1 -> Flag/1
  Constant/1 -> Count/1
  In1/1 -> Data/1

== system Control_test/InputProcessing/IBEOCANProcessing/IBEOSASProcessing/SAS1 Processing/ErrProcessing1/If Action Subsystem2 ==
  In1 : Inport
  In2 : Inport  Port=2
  Action Port : ActionPort  ActionType=elseif
  Add : Sum
  Constant : Constant  Value=0.02
  Constant1 : Constant
  Data : Outport
  Count : Outport  Port=2
  Flag : Outport  Port=3
  wires:
  Constant1/1 -> Flag/1
  Add/1 -> Count/1
  Constant/1 -> Add/2
  In2/1 -> Add/1
  In1/1 -> Data/1

== system Control_test/InputProcessing/IBEOCANProcessing/IBEOSASProcessing/SAS1 Processing/ErrProcessing2/If Action Subsystem ==
  In1 : Inport
  Action Port : ActionPort  ActionType=then
  Constant : Constant  Value=0
  Constant1 : Constant
  Data : Outport
  Count : Outport  Port=2
  Flag : Outport  Port=3
  wires:
  Constant/1 -> Data/1
  In1/1 -> Count/1
  Constant1/1 -> Flag/1

== system Control_test/InputProcessing/IBEOCANProcessing/IBEOSASProcessing/SAS1 Processing/ErrProcessing2/If Action Subsystem1 ==
  In1 : Inport
  Action Port : ActionPort  ActionType=else
  Constant : Constant  Value=0
  Constant1 : Constant  Value=0
  Data : Outport
  Count : Outport  Port=2
  Flag : Outport  Port=3
  wires:
  In1/1 -> Data/1
  Constant/1 -> Count/1
  Constant1/1 -> Flag/1

== system Control_test/InputProcessing/IBEOCANProcessing/IBEOSASProcessing/SAS1 Processing/ErrProcessing2/If Action Subsystem2 ==
  In1 : Inport
  In2 : Inport  Port=2
  Action Port : ActionPort  ActionType=elseif
  Add : Sum
  Constant : Constant  Value=0.02
  Constant1 : Constant
  Data : Outport
  Count : Outport  Port=2
  Flag : Outport  Port=3
  wires:
  In1/1 -> Data/1
  In2/1 -> Add/1
  Constant/1 -> Add/2
  Add/1 -> Count/1
  Constant1/1 -> Flag/1

== system Control_test/InputProcessing/VehicleCanProcessing/EMS1Processing/EMS1 Processing/ErrProcessing/If Action Subsystem ==
  In1 : Inport
  Action Port : ActionPort  ActionType=then
  Constant : Constant  Value=0
  Constant1 : Constant
  Data : Outport
  Count : Outport  Port=2
  Flag : Outport  Port=3
  wires:
  Constant1/1 -> Flag/1
  In1/1 -> Count/1
  Constant/1 -> Data/1

== system Control_test/InputProcessing/VehicleCanProcessing/EMS1Processing/EMS1 Processing/ErrProcessing/If Action Subsystem1 ==
  In1 : Inport
  Action Port : ActionPort  ActionType=else
  Constant : Constant  Value=0
  Constant1 : Constant  Value=0
  Data : Outport
  Count : Outport  Port=2
  Flag : Outport  Port=3
  wires:
  Constant1/1 -> Flag/1
  Constant/1 -> Count/1
  In1/1 -> Data/1

== system Control_test/InputProcessing/VehicleCanProcessing/EMS1Processing/EMS1 Processing/ErrProcessing/If Action Subsystem2 ==
  In1 : Inport
  In2 : Inport  Port=2
  Action Port : ActionPort  ActionType=elseif
  Add : Sum
  Constant : Constant  Value=0.02
  Constant1 : Constant
  Data : Outport
  Count : Outport  Port=2
  Flag : Outport  Port=3
  wires:
  Constant1/1 -> Flag/1
  Add/1 -> Count/1
  Constant/1 -> Add/2
  In2/1 -> Add/1
  In1/1 -> Data/1

== system Control_test/InputProcessing/VehicleCanProcessing/SAS1Processing/SAS1 Processing/ErrProcessing1/If Action Subsystem ==
  In1 : Inport
  Action Port : ActionPort  ActionType=then
  Constant : Constant  Value=0
  Constant1 : Constant
  Data : Outport
  Count : Outport  Port=2
  Flag : Outport  Port=3
  wires:
  Constant1/1 -> Flag/1
  In1/1 -> Count/1
  Constant/1 -> Data/1

== system Control_test/InputProcessing/VehicleCanProcessing/SAS1Processing/SAS1 Processing/ErrProcessing1/If Action Subsystem1 ==
  In1 : Inport
  Action Port : ActionPort  ActionType=else
  Constant : Constant  Value=0
  Constant1 : Constant  Value=0
  Data : Outport
  Count : Outport  Port=2
  Flag : Outport  Port=3
  wires:
  Constant1/1 -> Flag/1
  Constant/1 -> Count/1
  In1/1 -> Data/1

== system Control_test/InputProcessing/VehicleCanProcessing/SAS1Processing/SAS1 Processing/ErrProcessing1/If Action Subsystem2 ==
  In1 : Inport
  In2 : Inport  Port=2
  Action Port : ActionPort  ActionType=elseif
  Add : Sum
  Constant : Constant  Value=0.02
  Constant1 : Constant
  Data : Outport
  Count : Outport  Port=2
  Flag : Outport  Port=3
  wires:
  Constant1/1 -> Flag/1
  Add/1 -> Count/1
  Constant/1 -> Add/2
  In2/1 -> Add/1
  In1/1 -> Data/1

== system Control_test/InputProcessing/VehicleCanProcessing/SAS1Processing/SAS1 Processing/ErrProcessing2/If Action Subsystem ==
  In1 : Inport
  Action Port : ActionPort  ActionType=then
  Constant : Constant  Value=0
  Constant1 : Constant
  Data : Outport
  Count : Outport  Port=2
  Flag : Outport  Port=3
  wires:
  Constant/1 -> Data/1
  In1/1 -> Count/1
  Constant1/1 -> Flag/1

== system Control_test/InputProcessing/VehicleCanProcessing/SAS1Processing/SAS1 Processing/ErrProcessing2/If Action Subsystem1 ==
  In1 : Inport
  Action Port : ActionPort  ActionType=else
  Constant : Constant  Value=0
  Constant1 : Constant  Value=0
  Data : Outport
  Count : Outport  Port=2
  Flag : Outport  Port=3
  wires:
  In1/1 -> Data/1
  Constant/1 -> Count/1
  Constant1/1 -> Flag/1

== system Control_test/InputProcessing/VehicleCanProcessing/SAS1Processing/SAS1 Processing/ErrProcessing2/If Action Subsystem2 ==
  In1 : Inport
  In2 : Inport  Port=2
  Action Port : ActionPort  ActionType=elseif
  Add : Sum
  Constant : Constant  Value=0.02
  Constant1 : Constant
  Data : Outport
  Count : Outport  Port=2
  Flag : Outport  Port=3
  wires:
  In1/1 -> Data/1
  In2/1 -> Add/1
  Constant/1 -> Add/2
  Add/1 -> Count/1
  Constant1/1 -> Flag/1

== system Control_test/InputProcessing/VehicleCanProcessing/WhlSpdProcessing/WhlSpd Processing/ErrProcessing/If Action Subsystem ==
  In1 : Inport
  Action Port : ActionPort  ActionType=then
  Constant : Constant  Value=0
  Constant1 : Constant
  Data : Outport
  Count : Outport  Port=2
  Flag : Outport  Port=3
  wires:
  Constant1/1 -> Flag/1
  In1/1 -> Count/1
  Constant/1 -> Data/1

== system Control_test/InputProcessing/VehicleCanProcessing/WhlSpdProcessing/WhlSpd Processing/ErrProcessing/If Action Subsystem1 ==
  In1 : Inport
  Action Port : ActionPort  ActionType=else
  Constant : Constant  Value=0
  Constant1 : Constant  Value=0
  Data : Outport
  Count : Outport  Port=2
  Flag : Outport  Port=3
  wires:
  Constant1/1 -> Flag/1
  Constant/1 -> Count/1
  In1/1 -> Data/1

== system Control_test/InputProcessing/VehicleCanProcessing/WhlSpdProcessing/WhlSpd Processing/ErrProcessing/If Action Subsystem2 ==
  In1 : Inport
  In2 : Inport  Port=2
  Action Port : ActionPort  ActionType=elseif
  Add : Sum
  Constant : Constant  Value=0.02
  Constant1 : Constant
  Data : Outport
  Count : Outport  Port=2
  Flag : Outport  Port=3
  wires:
  Constant1/1 -> Flag/1
  Add/1 -> Count/1
  Constant/1 -> Add/2
  In2/1 -> Add/1
  In1/1 -> Data/1

== system Control_test/InputProcessing/VehicleCanProcessing/WhlSpdProcessing/WhlSpd Processing/ErrProcessing1/If Action Subsystem ==
  In1 : Inport
  Action Port : ActionPort  ActionType=then
  Constant : Constant  Value=0
  Constant1 : Constant
  Data : Outport
  Count : Outport  Port=2
  Flag : Outport  Port=3
  wires:
  Constant/1 -> Data/1
  In1/1 -> Count/1
  Constant1/1 -> Flag/1

== system Control_test/InputProcessing/VehicleCanProcessing/WhlSpdProcessing/WhlSpd Processing/ErrProcessing1/If Action Subsystem1 ==
  In1 : Inport
  Action Port : ActionPort  ActionType=else
  Constant : Constant  Value=0
  Constant1 : Constant  Value=0
  Data : Outport
  Count : Outport  Port=2
  Flag : Outport  Port=3
  wires:
  In1/1 -> Data/1
  Constant/1 -> Count/1
  Constant1/1 -> Flag/1

== system Control_test/InputProcessing/VehicleCanProcessing/WhlSpdProcessing/WhlSpd Processing/ErrProcessing1/If Action Subsystem2 ==
  In1 : Inport
  In2 : Inport  Port=2
  Action Port : ActionPort  ActionType=elseif
  Add : Sum
  Constant : Constant  Value=0.02
  Constant1 : Constant
  Data : Outport
  Count : Outport  Port=2
  Flag : Outport  Port=3
  wires:
  In1/1 -> Data/1
  In2/1 -> Add/1
  Constant/1 -> Add/2
  Add/1 -> Count/1
  Constant1/1 -> Flag/1

== system Control_test/InputProcessing/VehicleCanProcessing/WhlSpdProcessing/WhlSpd Processing/ErrProcessing2/If Action Subsystem ==
  In1 : Inport
  Action Port : ActionPort  ActionType=then
  Constant : Constant  Value=0
  Constant1 : Constant
  Data : Outport
  Count : Outport  Port=2
  Flag : Outport  Port=3
  wires:
  Constant1/1 -> Flag/1
  In1/1 -> Count/1
  Constant/1 -> Data/1

== system Control_test/InputProcessing/VehicleCanProcessing/WhlSpdProcessing/WhlSpd Processing/ErrProcessing2/If Action Subsystem1 ==
  In1 : Inport
  Action Port : ActionPort  ActionType=else
  Constant : Constant  Value=0
  Constant1 : Constant  Value=0
  Data : Outport
  Count : Outport  Port=2
  Flag : Outport  Port=3
  wires:
  Constant1/1 -> Flag/1
  Constant/1 -> Count/1
  In1/1 -> Data/1

== system Control_test/InputProcessing/VehicleCanProcessing/WhlSpdProcessing/WhlSpd Processing/ErrProcessing2/If Action Subsystem2 ==
  In1 : Inport
  In2 : Inport  Port=2
  Action Port : ActionPort  ActionType=elseif
  Add : Sum
  Constant : Constant  Value=0.02
  Constant1 : Constant
  Data : Outport
  Count : Outport  Port=2
  Flag : Outport  Port=3
  wires:
  Constant1/1 -> Flag/1
  Add/1 -> Count/1
  Constant/1 -> Add/2
  In2/1 -> Add/1
  In1/1 -> Data/1

== system Control_test/InputProcessing/VehicleCanProcessing/WhlSpdProcessing/WhlSpd Processing/ErrProcessing3/If Action Subsystem ==
  In1 : Inport
  Action Port : ActionPort  ActionType=then
  Constant : Constant  Value=0
  Constant1 : Constant
  Data : Outport
  Count : Outport  Port=2
  Flag : Outport  Port=3
  wires:
  Constant/1 -> Data/1
  In1/1 -> Count/1
  Constant1/1 -> Flag/1

== system Control_test/InputProcessing/VehicleCanProcessing/WhlSpdProcessing/WhlSpd Processing/ErrProcessing3/If Action Subsystem1 ==
  In1 : Inport
  Action Port : ActionPort  ActionType=else
  Constant : Constant  Value=0
  Constant1 : Constant  Value=0
  Data : Outport
  Count : Outport  Port=2
  Flag : Outport  Port=3
  wires:
  In1/1 -> Data/1
  Constant/1 -> Count/1
  Constant1/1 -> Flag/1

== system Control_test/InputProcessing/VehicleCanProcessing/WhlSpdProcessing/WhlSpd Processing/ErrProcessing3/If Action Subsystem2 ==
  In1 : Inport
  In2 : Inport  Port=2
  Action Port : ActionPort  ActionType=elseif
  Add : Sum
  Constant : Constant  Value=0.02
  Constant1 : Constant
  Data : Outport
  Count : Outport  Port=2
  Flag : Outport  Port=3
  wires:
  In1/1 -> Data/1
  In2/1 -> Add/1
  Constant/1 -> Add/2
  Add/1 -> Count/1
  Constant1/1 -> Flag/1

== system Control_test/OutputProcessing/VehicleCanProcessing/LKAS2/Angle 2 Torque/PI controller/SAS_Control ==
  SAS_Cmd : Inport
  SAS : Inport  Port=2
  ActiveFlag : Inport  Port=3
  P_gain_sas1 : Inport  Port=4
  Add : Sum  Inputs=+++
  Angle_gain : Gain  Gain=0.001
  Gain : Gain
  Gain1 : Gain  Gain=1/3
  Integer Delay : Delay  DelayLength=1
  Integer Delay1 : Delay
  Integer Delay2 : Delay  DelayLength=1
  Product1 : Product  RndMeth=Zero
  Product2 : Product  RndMeth=Zero
  SAS_Saturation1 : Saturate  UpperLimit=2.5  LowerLimit=-2.5
  SAS_Saturation1_old : Saturate  UpperLimit=0.75  LowerLimit=-0.75
  SAS_Saturation2 : Saturate  UpperLimit=20  LowerLimit=-20
  SAS_Saturation2_old : Saturate  UpperLimit=5  LowerLimit=-5
  Sum : Sum  Inputs=|+-
  Sum1 : Sum  Inputs=|+-
  Sum2 : Sum  Inputs=|+-
  Terminator : Terminator
  Terminator1 : Terminator
  SAS_Speed_error : Outport
  wires:
  SAS_Cmd/1 -> Sum/1
  SAS/1 -> Sum/2, Integer Delay/1, Sum1/1
  P_gain_sas1/1 -> Angle_gain/1
  Sum2/1 -> SAS_Saturation2_old/1, SAS_Saturation2/1
  Product2/1 -> Sum2/1
  ActiveFlag/1 -> Product2/2
  Product1/1 -> SAS_Saturation1_old/1, SAS_Saturation1/1
  Integer Delay/1 -> Sum1/2
  Sum1/1 -> Gain/1
  Angle_gain/1 -> Product1/2
  Sum/1 -> Product1/1
  Integer Delay1/1 -> Add/2
  Integer Delay2/1 -> Add/3
  Add/1 -> Gain1/1
  Gain/1 -> Add/1, Integer Delay1/1, Integer Delay2/1
  Gain1/1 -> Sum2/2
  SAS_Saturation1_old/1 -> Product2/1  "SAS_sat1"
  SAS_Saturation2_old/1 -> SAS_Speed_error/1  "SAS_sat2"
  SAS_Saturation1/1 -> Terminator/1
  SAS_Saturation2/1 -> Terminator1/1

== system Control_test/OutputProcessing/VehicleCanProcessing/LKAS2/Angle 2 Torque/PI controller/SAS_Speed_Control ==
  speed err : Inport
  P_gain_spd1 : Inport  Port=2
  I_gain_spd1 : Inport  Port=3
  Active_Flag : Inport  Port=4
  Compare To Zero : simulink/Logic and Bit Operations/Compare To Zero  relop===  OutDataTypeStr=uint8  ZeroCross=off
  Discrete-Time Integrator : DiscreteIntegrator  ExternalReset=level  SampleTime=-1  LimitOutput=on  UpperSaturationLimit=1000  LowerSaturationLimit=-1000
  Gain1 : Gain  Gain=327.68
  Gain2 : Gain  Gain=1/255
  Gain3 : Gain  Gain=1/255
  Goto1 : Goto  Commented=on  GotoTag=P_Ctl_Out_old
  Goto2 : Goto  Commented=on  GotoTag=I_Ctl_Out_old
  Product5 : Product  RndMeth=Zero
  Product7 : Product  RndMeth=Zero
  SASSpeedSat1 : Saturate  UpperLimit=2000  LowerLimit=-2000
  SASSpeedSat1_old : Saturate  UpperLimit=250  LowerLimit=-250
  SASSpeedSat2 : Saturate  UpperLimit=7.5  LowerLimit=-7.5
  SASSpeedSat2_old : Saturate  UpperLimit=4  LowerLimit=-4
  Sum3 : Sum
  Terminator : Terminator
  Terminator1 : Terminator
  Out1 : Outport
  wires:
  Sum3/1 -> Gain3/1
  SASSpeedSat2_old/1 -> Out1/1  "SASSpeed_sat2"
  Gain3/1 -> SASSpeedSat2_old/1, SASSpeedSat2/1
  Gain2/1 -> Product7/1
  Gain1/1 -> Discrete-Time Integrator/1
  Discrete-Time Integrator/1 -> Gain2/1
  Product7/1 -> Sum3/2, Goto2/1  "I_value"
  Active_Flag/1 -> Compare To Zero/1
  Compare To Zero/1 -> Discrete-Time Integrator/2
  SASSpeedSat1_old/1 -> Sum3/1, Goto1/1  "SASSpeed_sat1"
  Product5/1 -> SASSpeedSat1_old/1, SASSpeedSat1/1  "P_value"
  P_gain_spd1/1 -> Product5/2
  I_gain_spd1/1 -> Product7/2
  speed err/1 -> Product5/1, Gain1/1
  SASSpeedSat1/1 -> Terminator/1
  SASSpeedSat2/1 -> Terminator1/1

== system Control_test/OutputProcessing/VehicleCanProcessing/LKAS2/TxLKAS2CAN/MessageCounter/Shinho Systems Co., Ltd. ==
  note: Director : Kyu hoon, Lee
      |
      | Shinho Systems Co., Ltd.
      | Tel : +82-31-737-6800
      | Fax : +82-31-737-6809
      |
      | 2009. 6. 18.
  Model Info : Subsystem  LoadFcn=slcm LoadBlock;  InitFcn=slcm('UpdateAllCMBlocksInThisModelInit')  mask(CMBlock){InitialSaveTempField=, InitialBlockCM=, BlockCM=None, Frame=on, SaveTempField=, DisplayStringWithTags=|, MaskDisplayString=Model Info\nWed Nov 07 03:44:04 2012\n\n\nMPC\n06-Apr-2016 16:52:46\n\n1.3565, HorizontalTextAlignment=Center, LeftAlignmentValue=0.5, SourceBlockDiagram=Control_test, TagMaxNumber=20, CMTag1=, CMTag2=, CMTag3=, CMTag4=, CMTag5=, CMTag6=, CMTag7=, CMTag8=, CMTag9=, CMTag10=, CMTag11=, CMTag12=, CMTag13=, CMTag14=, CMTag15=, CMTag16=, CMTag17=, CMTag18=, CMTag19=, CMTag20=}
      mask DisplayStringWithTags=|
      | Model Info
      | %<Created>
      |
      |
      | %<LastModifiedBy>
      | %<LastModificationDate>
      |
      | %<ModelVersion>
      mask help: This block allows revision control information to be displayed within the model.
      settings: CopyFcn=slcm CopyBlock;  DeleteFcn=slcm Cancel;  PostSaveFcn=slcm('UpdateAllCMBlocksInThisModel')  NameChangeFcn=slcm Rename;  OpenFcn=slcm
      mask Display: text(str2num(LeftAlignmentValue), 0.5, MaskDisplayString, 'HorizontalAlignment', HorizontalTextAlignment)
